simulink model "CartPole"  (R2022b)
settings: Solver=FixedStepAuto  StartTime=0.0  StopTime=20  FixedStep=0.01  RelTol=1e-3
values from neighbouring files (symbols this model uses):
  g = 9.81    [startup.m]
  L = 1    [startup.m]
  M = cL*cH*0.1*rho_aluminum    (= 16.26)    [startup.m]
  m = L*(0.05)*(0.05)*rho_aluminum    (= 6.775)    [startup.m]
  theta_0 = deg2rad(20)    [startup.m]
  x_0 = 0    [startup.m]
undefined symbols (not defined in the file or in its folder): K
settings Model: Creator=logan  LastModifiedBy=logan

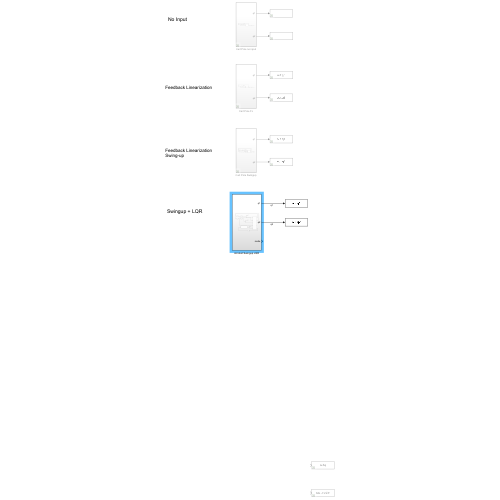
[thumbnail: Simulink's stored preview of the top-level diagram]
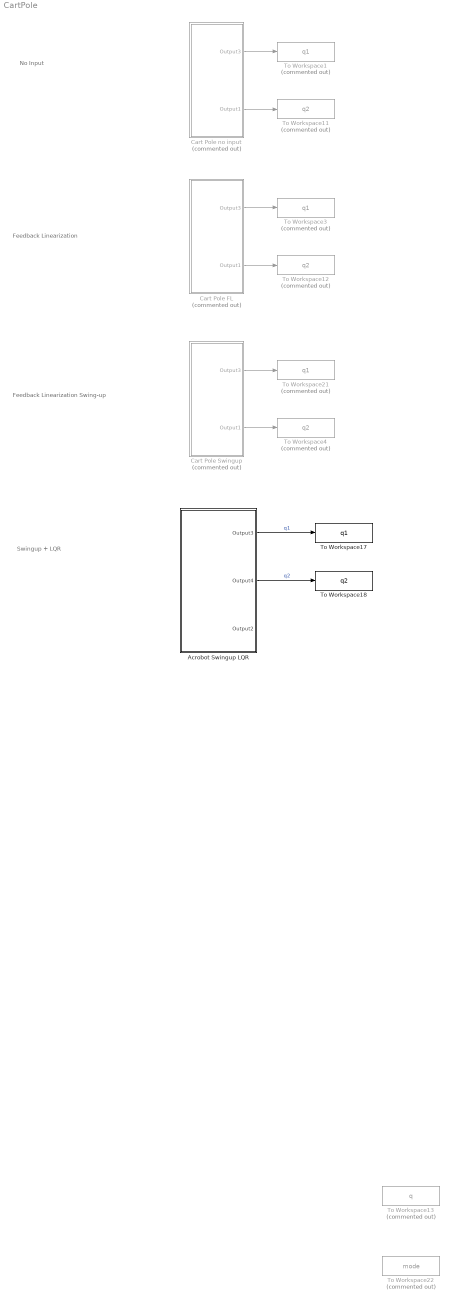
== system CartPole ==
  note: Feedback Linearization
  note: No Input
  note: Feedback Linearization
      | Swing-up
  note: Swingup + LQR
  Acrobot Swingup LQR : Subsystem
  Cart Pole FL : Subsystem  Commented=on
  Cart Pole Swingup : Subsystem  Commented=on
  Cart Pole no input : Subsystem  Commented=on
  To Workspace1 : ToWorkspace  Commented=on  VariableName=q1  SaveFormat=Timeseries  SampleTime=-1
  To Workspace11 : ToWorkspace  Commented=on  VariableName=q2  SaveFormat=Timeseries  SampleTime=-1
  To Workspace12 : ToWorkspace  Commented=on  VariableName=q2  SaveFormat=Timeseries  SampleTime=-1
  To Workspace13 : ToWorkspace  Commented=on  VariableName=q  SaveFormat=Timeseries  SampleTime=-1
  To Workspace17 : ToWorkspace  VariableName=q1  SaveFormat=Timeseries  SampleTime=-1
  To Workspace18 : ToWorkspace  VariableName=q2  SaveFormat=Timeseries  SampleTime=-1
  To Workspace21 : ToWorkspace  Commented=on  VariableName=q1  SaveFormat=Timeseries  SampleTime=-1
  To Workspace22 : ToWorkspace  Commented=on  VariableName=mode  SaveFormat=Timeseries  SampleTime=-1
  To Workspace3 : ToWorkspace  Commented=on  VariableName=q1  SaveFormat=Timeseries  SampleTime=-1
  To Workspace4 : ToWorkspace  Commented=on  VariableName=q2  SaveFormat=Timeseries  SampleTime=-1
  wires:
  Cart Pole no input/1(Output3) -> To Workspace1/1
  Cart Pole no input/2(Output1) -> To Workspace11/1
  Cart Pole FL/2(Output1) -> To Workspace12/1
  Cart Pole FL/1(Output3) -> To Workspace3/1
  Cart Pole Swingup/1(Output3) -> To Workspace21/1
  Cart Pole Swingup/2(Output1) -> To Workspace4/1
  Acrobot Swingup LQR/2(Output4) -> To Workspace18/1  "q2"
  Acrobot Swingup LQR/1(Output3) -> To Workspace17/1  "q1"

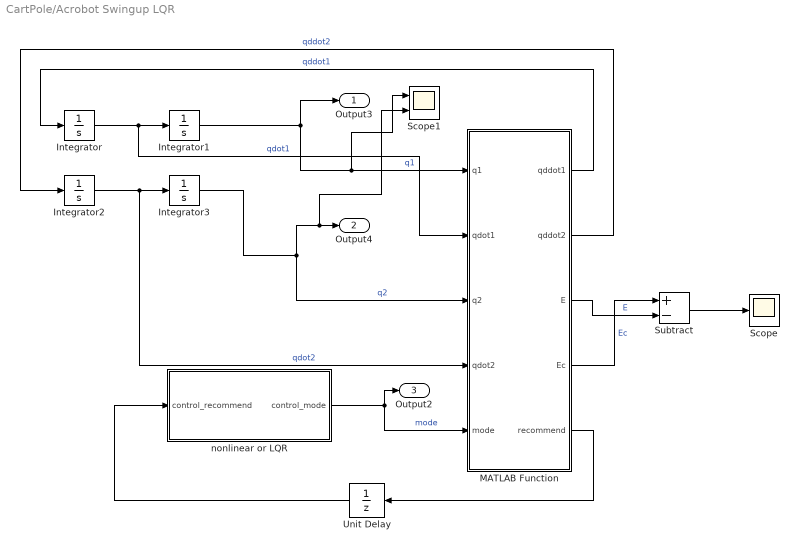
== system CartPole/Acrobot Swingup LQR ==
  Integrator : Integrator
  Integrator1 : Integrator  InitialCondition=theta_0
  Integrator2 : Integrator
  Integrator3 : Integrator  InitialCondition=x_0
  MATLAB Function : MATLAB Function  TreatAsAtomicUnit=on
  Scope : Scope
  Scope1 : Scope  NumInputPorts=2
  Subtract : Sum  Inputs=+-
  Unit Delay : UnitDelay  SampleTime=.01  HasFrameUpgradeWarning=on
  nonlinear or LQR : Stateflow chart  TreatAsAtomicUnit=on
  Output3 : Outport
  Output4 : Outport  Port=2
  Output2 : Outport  Port=3
  wires:
  Integrator/1 -> MATLAB Function/2(qdot1), Integrator1/1  "qdot1"
  Integrator1/1 -> Output3/1, Scope1/1, MATLAB Function/1(q1)  "q1"
  Integrator2/1 -> MATLAB Function/4(qdot2), Integrator3/1  "qdot2"
  MATLAB Function/2(qddot2) -> Integrator2/1  "qddot2"
  Integrator3/1 -> Scope1/2, Output4/1, MATLAB Function/3(q2)  "q2"
  MATLAB Function/1(qddot1) -> Integrator/1  "qddot1"
  nonlinear or LQR/1(control_mode) -> MATLAB Function/5(mode), Output2/1  "mode"
  MATLAB Function/5(recommend) -> Unit Delay/1
  Unit Delay/1 -> nonlinear or LQR/1(control_recommend)
  MATLAB Function/4(Ec) -> Subtract/1  "Ec"
  MATLAB Function/3(E) -> Subtract/2  "E"
  Subtract/1 -> Scope/1

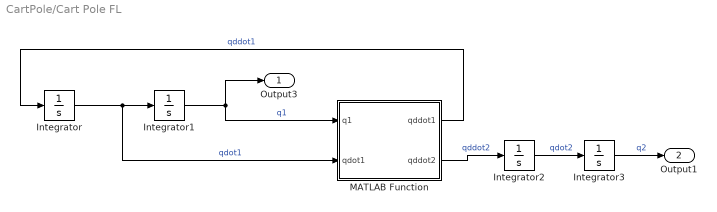
== system CartPole/Cart Pole FL ==
  Integrator : Integrator
  Integrator1 : Integrator  InitialCondition=theta_0
  Integrator2 : Integrator
  Integrator3 : Integrator  InitialCondition=x_0
  MATLAB Function : MATLAB Function  TreatAsAtomicUnit=on
  Output3 : Outport
  Output1 : Outport  Port=2
  wires:
  Integrator/1 -> MATLAB Function/2(qdot1), Integrator1/1  "qdot1"
  MATLAB Function/1(qddot1) -> Integrator/1  "qddot1"
  Integrator1/1 -> MATLAB Function/1(q1), Output3/1  "q1"
  MATLAB Function/2(qddot2) -> Integrator2/1  "qddot2"
  Integrator2/1 -> Integrator3/1  "qdot2"
  Integrator3/1 -> Output1/1  "q2"

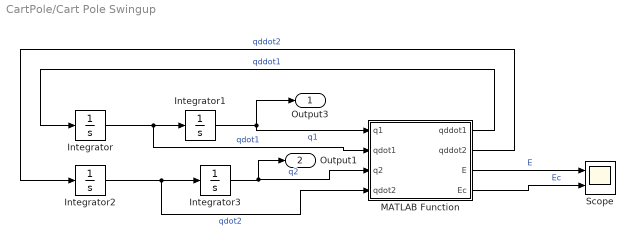
== system CartPole/Cart Pole Swingup ==
  Integrator : Integrator
  Integrator1 : Integrator  InitialCondition=theta_0
  Integrator2 : Integrator
  Integrator3 : Integrator  InitialCondition=x_0
  MATLAB Function : MATLAB Function  TreatAsAtomicUnit=on
  Scope : Scope  NumInputPorts=2
  Output3 : Outport
  Output1 : Outport  Port=2
  wires:
  Integrator/1 -> MATLAB Function/2(qdot1), Integrator1/1  "qdot1"
  MATLAB Function/1(qddot1) -> Integrator/1  "qddot1"
  Integrator1/1 -> MATLAB Function/1(q1), Output3/1  "q1"
  MATLAB Function/2(qddot2) -> Integrator2/1  "qddot2"
  Integrator2/1 -> MATLAB Function/4(qdot2), Integrator3/1  "qdot2"
  Integrator3/1 -> MATLAB Function/3(q2), Output1/1  "q2"
  MATLAB Function/3(E) -> Scope/1  "E"
  MATLAB Function/4(Ec) -> Scope/2  "Ec"

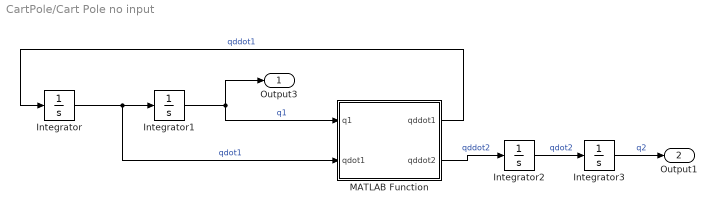
== system CartPole/Cart Pole no input ==
  Integrator : Integrator
  Integrator1 : Integrator  InitialCondition=theta_0
  Integrator2 : Integrator
  Integrator3 : Integrator  InitialCondition=x_0
  MATLAB Function : MATLAB Function  TreatAsAtomicUnit=on
  Output3 : Outport
  Output1 : Outport  Port=2
  wires:
  Integrator/1 -> MATLAB Function/2(qdot1), Integrator1/1  "qdot1"
  MATLAB Function/1(qddot1) -> Integrator/1  "qddot1"
  Integrator1/1 -> MATLAB Function/1(q1), Output3/1  "q1"
  MATLAB Function/2(qddot2) -> Integrator2/1  "qddot2"
  Integrator2/1 -> Integrator3/1  "qdot2"
  Integrator3/1 -> Output1/1  "q2"

== stateflow chart CartPole/Acrobot Swingup LQR/nonlinear or LQR ==
  state nonlinear
    control_mode=1;
  state LQR
    control_mode=2;
  (default) -> nonlinear
  nonlinear -> LQR : [control_recommend==2]
  data: control_recommend input; control_mode output

== matlab function CartPole/Acrobot Swingup LQR/MATLAB Function ==
  data: q1 input; qdot1 input; q2 input; qdot2 input; mode input; g parameter; qddot1 output; qddot2 output; M parameter; L parameter; E output; Ec output; recommend output; m parameter; K parameter
function [qddot1,qddot2,E,Ec,recommend] = EoM(q1,qdot1,q2,qdot2,mode,g,M,L,m,K)

m11 = 1/3*m*L^2;
m12 = 1/2*m*L*cos(q1);
m22 = M+m;

phi1 = -1/2*m*g*L*sin(q1);
h2 = -1/2*m*L*qdot1^2*sin(q1);

m22_bar = m22 - m12^2/m11;
phi_bar = -1/m11*phi1;
h_bar = h2;

% energy of pendulum
I = 1/3*m*L^2;
E = 1/2*I*qdot1^2 + m*g*L/2*cos(q1);
Ec = m*g*L/2;

% swing-up controller
u_nonlinear = (E-Ec)*qdot1*cos(q1) - 21*q2 - 10*qdot2;
F_nonlinear = u_nonlinear + h_bar + phi_bar;

% % LQR
z1 = wrapToPi(q1);
F_lqr = -K*[z1; q2; qdot1; qdot2];

% controller selection
if mode == 1
    F = F_nonlinear;
else
    F = F_lqr;
end

% dynamics
qddot2 = 1/m22_bar*(F - h_bar - phi_bar);
qddot1 = -1/m11*(phi1 + m12*qddot2);

% starts in nonlinear mode, switches to LQR at the right moment
% does not switch back to nonlinear mode once we are in LQR
z1 = wrapToPi(q1);
if abs(z1) < deg2rad(5)
    recommend = 2; % LQR
else
    recommend = 1; % nonlinear
end

== matlab function CartPole/Cart Pole no input/MATLAB Function ==
  data: qddot1 output; q1 input; qdot1 input; g parameter; m parameter; L parameter; qddot2 output; M parameter
function [qddot1, qddot2]   = EoM(q1,qdot1,g,m,L,M)

m22_bar = M + m*(1 - 3/4*cos(q1)^2);
h2_bar = 1/2*m*L*qdot1^2*sin(q1);
phi2_bar = -3/4*m*g*sin(q1)*cos(q1);

% dynamics
F = 0;
qddot2 = 1/m22_bar*(F + h2_bar + phi2_bar);
qddot1 = 3/(2*L)*(g*sin(q1)-qddot2*cos(q1));

== matlab function CartPole/Cart Pole Swingup/MATLAB Function ==
  data: qddot1 output; q1 input; qdot1 input; q2 input; qdot2 input; g parameter; m parameter; qddot2 output; M parameter; L parameter; E output; Ec output
function [qddot1,qddot2,E,Ec]   = EoM(q1,qdot1,q2,qdot2,g,m,M, L)

m22_bar = M + m*(1 - 3/4*cos(q1)^2);
h2_bar = 1/2*m*L*qdot1^2*sin(q1);
phi2_bar = -3/4*m*g*sin(q1)*cos(q1);

% energy of pendulum
I = 1/3*m*L^2;
E = 1/2*I*qdot1^2 + m*g*L/2*cos(q1);
Ec = m*g*L/2;

% dynamics
u = (E-Ec)*qdot1*cos(q1) - 21*q2 - 10*qdot2;
F = u - h2_bar - phi2_bar;
qddot2 = 1/m22_bar*(F + h2_bar + phi2_bar);
qddot1 = 3/(2*L)*(g*sin(q1)-qddot2*cos(q1));

== matlab function CartPole/Cart Pole FL/MATLAB Function ==
  data: qddot1 output; q1 input; qdot1 input; g parameter; m parameter; L parameter; qddot2 output; M parameter
function [qddot1, qddot2]   = EoM(q1,qdot1,g,m,L,M)

m22_bar = M + m*(1 - 3/4*cos(q1)^2);
h2_bar = 1/2*m*L*qdot1^2*sin(q1);
phi2_bar = -3/4*m*g*sin(q1)*cos(q1);

% dynamics
u = 0;
F = u - h2_bar - phi2_bar;
qddot2 = 1/m22_bar*(F + h2_bar + phi2_bar);
qddot1 = 3/(2*L)*(g*sin(q1)-qddot2*cos(q1));
